simulink subsystem "MovimientoWilly"  (R2021b)
settings: Solver=VariableStepAuto  StartTime=0.0  StopTime=10.0  RelTol=1e-3
settings Model: Creator=yo  LastModifiedBy=yo

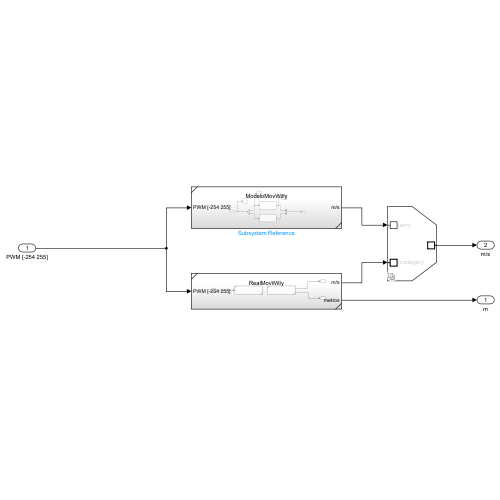
[thumbnail: Simulink's stored preview of the top-level diagram]
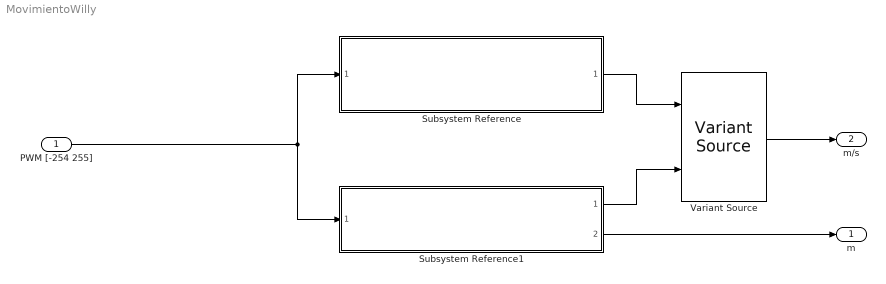
== system MovimientoWilly ==
  PWM [-254 255] : Inport
  Subsystem Reference : Subsystem  ReferencedSubsystem=ModeloMovWilly
  Subsystem Reference1 : Subsystem  ReferencedSubsystem=RealMovWilly
  Variant Source : VariantSource  VariantControlMode=sim codegen switching  ShowConditionOnBlock=on
  m : Outport
  m/s : Outport  Port=2
  wires:
  PWM [-254 255]/1 -> Subsystem Reference/1, Subsystem Reference1/1
  Subsystem Reference/1 -> Variant Source/1
  Subsystem Reference1/1 -> Variant Source/2
  Variant Source/1 -> m/s/1
  Subsystem Reference1/2 -> m/1
